simulink model "Part2og"  (R2019b)
settings: Solver=VariableStepAuto  StartTime=0.0  StopTime=10.0  RelTol=1e-3
settings Model: Creator=jingl  LastModifiedBy=TimRo
settings SFSimCC: CustomCodeUndefinedFunction=UseInterfaceOnly

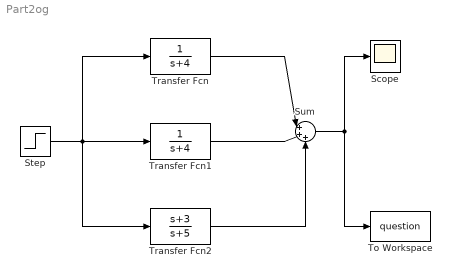
== system Part2og ==
  Scope : Scope
  Step : Step  Time=0  SampleTime=0
  Sum : Sum  Inputs=|+++
  To Workspace : ToWorkspace  VariableName=question  SaveFormat=Timeseries  SampleTime=-1
  Transfer Fcn : TransferFcn  Denominator=[1 4]
  Transfer Fcn1 : TransferFcn  Denominator=[1 4]
  Transfer Fcn2 : TransferFcn  Numerator=[1 3]  Denominator=[1 5]
  wires:
  Step/1 -> Transfer Fcn2/1, Transfer Fcn/1, Transfer Fcn1/1
  Sum/1 -> To Workspace/1, Scope/1
  Transfer Fcn2/1 -> Sum/3
  Transfer Fcn1/1 -> Sum/2
  Transfer Fcn/1 -> Sum/1
